simulink model "balancingOptTauExternalFsmForStep"  (Simulink 8.3)
settings: Solver=FixedStepDiscrete  StartTime=0.0  StopTime=simulationTime  FixedStep=Ts  RelTol=1e-3
InitFcn:
  | initBalancingOptTauExternalFsmForStep;
values from neighbouring files (symbols this model uses):
  localName = 'matlabTorqueBalancing'    [initBalancingOptTauExternalFsmForStep.m]
  Ts = 0.01    [initBalancingOptTauExternalFsmForStep.m]
undefined symbols (not defined in the file or in its folder): dampings, DiscIntNeverNeededParam, forceThreshold, gainMomentum, gainsDCOM, gainsICOM, gainsPCOM, impedances, impedencesSat, increasingRatesImp, qTildeMax, ROBOT_DOF_FOR_SIMULINK
undefined symbols (not defined in the file): robotName
libraries: WBCLibrary x45
settings Model: Creator=daniele  LastModifiedBy=daniele
settings DataIOCC: SignalLoggingSaveFormat=Dataset
settings OptimizationCC: ExpressionDepthLimit=2147483647
settings DebuggingCC: FcnCallInpInsideContextMsg=EnableAllAsWarning
settings SFSimCC: SimParseCustomCode=off

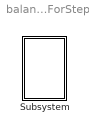
== system balancingOptTauExternalFsmForStep ==
  Subsystem : Subsystem  mask{robotName=robotName, Ts=Ts, localName=localName}
      mask prompts: robotName "robot name"; localName "module name"

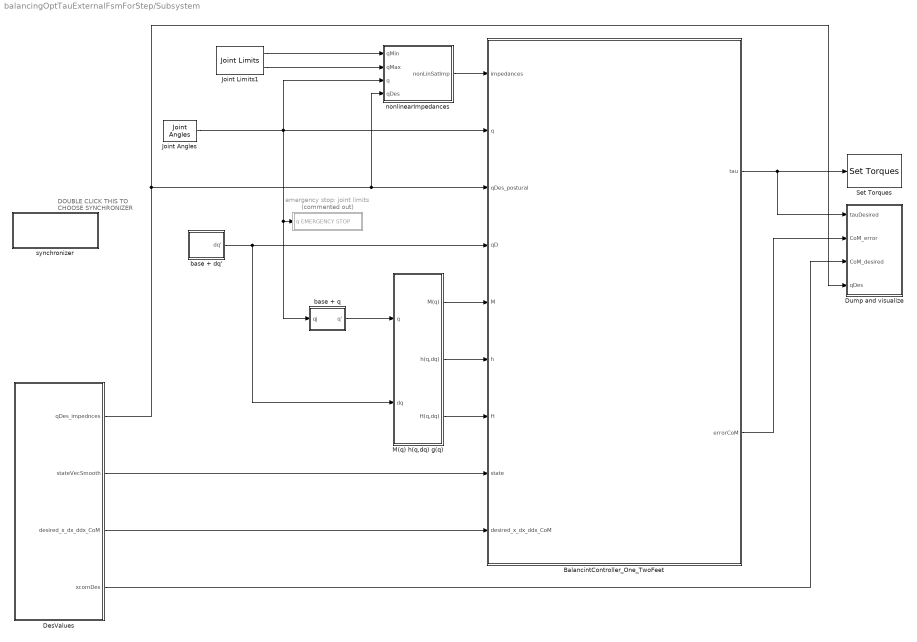
== system balancingOptTauExternalFsmForStep/Subsystem ==
  note: DOUBLE CLICK THIS TO
      |  CHOOSE SYNCHRONIZER
  BalancintController_One_TwoFeet : Subsystem
  DesValues : Subsystem
  Dump and visualize : Subsystem
  Joint Angles : WBCLibrary/wholeBodyStates/Joint Angles  robotName=robotName  localName=localName
  Joint Limits1 : WBCLibrary/wholeBodyModel/Joint Limits  robotName=robotName  localName=localName
  M(q) h(q,dq) g(q) : Subsystem
  Set Torques : WBCLibrary/wholeBodyActuators/Set Torques  val=6  robotName=robotName  localName=localName
  base + dq' : Subsystem
  base + q : Subsystem
  emergency stop: joint limits : Subsystem  Commented=on
  nonlinearImpedances : Subsystem
  synchronizer : Subsystem
  wires:
  base + q/1(q') -> M(q) h(q,dq) g(q)/1(q)
  M(q) h(q,dq) g(q)/3(H(q,dq)) -> BalancintController_One_TwoFeet/7(H)
  base + dq'/1(dq') -> M(q) h(q,dq) g(q)/2(dq), BalancintController_One_TwoFeet/4(qD)
  M(q) h(q,dq) g(q)/1(M(q)) -> BalancintController_One_TwoFeet/5(M)
  M(q) h(q,dq) g(q)/2(h(q,dq)) -> BalancintController_One_TwoFeet/6(h)
  BalancintController_One_TwoFeet/1(tau) -> Set Torques/1, Dump and visualize/1(tauDesired)
  BalancintController_One_TwoFeet/2(errorCoM) -> Dump and visualize/2(CoM_error)
  DesValues/4(xcomDes) -> Dump and visualize/3(CoM_desired)
  DesValues/3(desired_x_dx_ddx_CoM) -> BalancintController_One_TwoFeet/9(desired_x_dx_ddx_CoM)
  nonlinearImpedances/1(nonLinSatImp) -> BalancintController_One_TwoFeet/1(impedances)
  DesValues/2(stateVecSmooth) -> BalancintController_One_TwoFeet/8(state)
  DesValues/1(qDes_impednces) -> Dump and visualize/4(qDes), nonlinearImpedances/4(qDes), BalancintController_One_TwoFeet/3(qDes_postural)
  Joint Limits1/1 -> nonlinearImpedances/1(qMin)
  Joint Limits1/2 -> nonlinearImpedances/2(qMax)
  Joint Angles/1 -> nonlinearImpedances/3(q), base + q/1(qj), emergency stop: joint limits/1(q EMERGENCY STOP), BalancintController_One_TwoFeet/2(q)

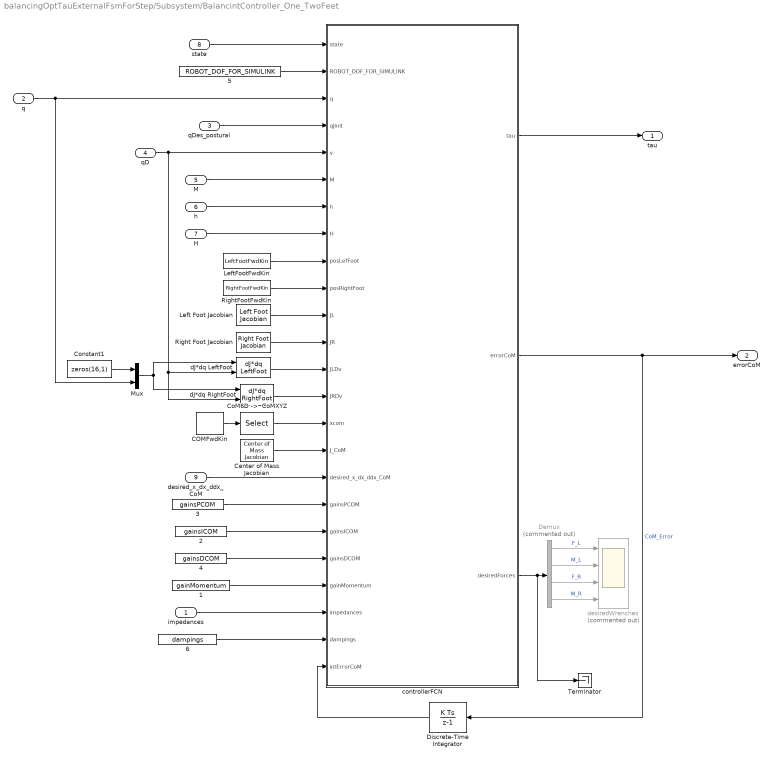
== system balancingOptTauExternalFsmForStep/Subsystem/BalancintController_One_TwoFeet ==
  impedances : Inport
  q : Inport  Port=2
  qDes_postural : Inport  Port=3
  qD : Inport  Port=4
  M : Inport  Port=5
  h : Inport  Port=6
  H : Inport  Port=7
  state : Inport  Port=8
  desired_x_dx_ddx_CoM : Inport  Port=9
  "    1" : Constant  Value=gainMomentum
  "    2" : Constant  Value=gainsICOM
  "    3" : Constant  Value=gainsPCOM
  "    4" : Constant  Value=gainsDCOM
  "    5" : Constant  Value=ROBOT_DOF_FOR_SIMULINK
  "    6" : Constant  Value=dampings
  "COMFwdKin " : WBCLibrary/wholeBodyModel/Forward Kinematics/COMFwdKin   robotName=robotName  localName=localName
  Center of Mass Jacobian : WBCLibrary/wholeBodyModel/Jacobians/Center of Mass Jacobian  robotName=robotName  localName=localName
  "CoM6D ->  CoMXYZ" : Selector  InputPortWidth=7  Indices=[1 2 3]
  Constant1 : Constant  Value=zeros(16,1)
  Demux : Demux  Commented=on
  Discrete-Time Integrator : DiscreteIntegrator  InitialCondition=[0 0 0]  SampleTime=Ts  ICPrevOutput=DiscIntNeverNeededParam  ICPrevScaledInput=DiscIntNeverNeededParam
  Left Foot Jacobian : WBCLibrary/wholeBodyModel/Jacobians/Left Foot Jacobian  robotName=robotName  localName=localName
  LeftFootFwdKin : WBCLibrary/wholeBodyModel/Forward Kinematics/LeftFootFwdKin  robotName=robotName  localName=localName
  Mux : Mux  Inputs=2
  Right Foot Jacobian : WBCLibrary/wholeBodyModel/Jacobians/Right Foot Jacobian  robotName=robotName  localName=localName
  RightFootFwdKin : WBCLibrary/wholeBodyModel/Forward Kinematics/RightFootFwdKin  robotName=robotName  localName=localName
  Terminator : Terminator
  controllerFCN : MATLAB Function  TreatAsAtomicUnit=on
  dJ*dq LeftFoot : WBCLibrary/wholeBodyModel/Dynamics/dJ*dq LeftFoot  val=9  robotName=robotName  localName=localName
  dJ*dq RightFoot : WBCLibrary/wholeBodyModel/Dynamics/dJ*dq RightFoot  val=9  robotName=robotName  localName=localName
  desiredWrenches : Scope  Commented=on  NumInputPorts=4
      settings: ShowLegends=on  TimeRange=150  YMin=-5~-5~63.70967741935465~-5  YMax=5~5~150~5  SaveName=ScopeData2
  tau : Outport
  errorCoM : Outport  Port=2
  wires:
  q/1 -> Mux/2, controllerFCN/3(q)
  qDes_postural/1 -> controllerFCN/4(qjInit)
  qD/1 -> dJ*dq RightFoot/2, dJ*dq LeftFoot/2, controllerFCN/5(v)
  M/1 -> controllerFCN/6(M)
  h/1 -> controllerFCN/7(h)
  H/1 -> controllerFCN/8(H)
  Left Foot Jacobian/1 -> controllerFCN/11(JL)
  Right Foot Jacobian/1 -> controllerFCN/12(JR)
  desired_x_dx_ddx_CoM/1 -> controllerFCN/17(desired_x_dx_ddx_CoM)
  impedances/1 -> controllerFCN/22(impedances)
  Discrete-Time Integrator/1 -> controllerFCN/24(intErrorCoM)
  "    3"/1 -> controllerFCN/18(gainsPCOM)
  "    1"/1 -> controllerFCN/21(gainMomentum)
  "    2"/1 -> controllerFCN/19(gainsICOM)
  "    4"/1 -> controllerFCN/20(gainsDCOM)
  controllerFCN/1(tau) -> tau/1
  "    5"/1 -> controllerFCN/2(ROBOT_DOF_FOR_SIMULINK)
  "    6"/1 -> controllerFCN/23(dampings)
  controllerFCN/3(desiredForces) -> Terminator/1, Demux/1
  Demux/1 -> desiredWrenches/1  "F_L"
  Demux/2 -> desiredWrenches/2  "M_L"
  Demux/3 -> desiredWrenches/3  "F_R"
  Demux/4 -> desiredWrenches/4  "M_R"
  state/1 -> controllerFCN/1(state)
  dJ*dq LeftFoot/1 -> controllerFCN/13(JLDv)
  dJ*dq RightFoot/1 -> controllerFCN/14(JRDv)
  Constant1/1 -> Mux/1
  Mux/1 -> dJ*dq RightFoot/1, dJ*dq LeftFoot/1
  "COMFwdKin "/1 -> "CoM6D ->  CoMXYZ"/1
  "CoM6D ->  CoMXYZ"/1 -> controllerFCN/15(xcom)
  RightFootFwdKin/1 -> controllerFCN/10(posRightFoot)
  Center of Mass Jacobian/1 -> controllerFCN/16(J_CoM)
  LeftFootFwdKin/1 -> controllerFCN/9(posLefFoot)
  controllerFCN/2(errorCoM) -> Discrete-Time Integrator/1, errorCoM/1  "CoM_Error"

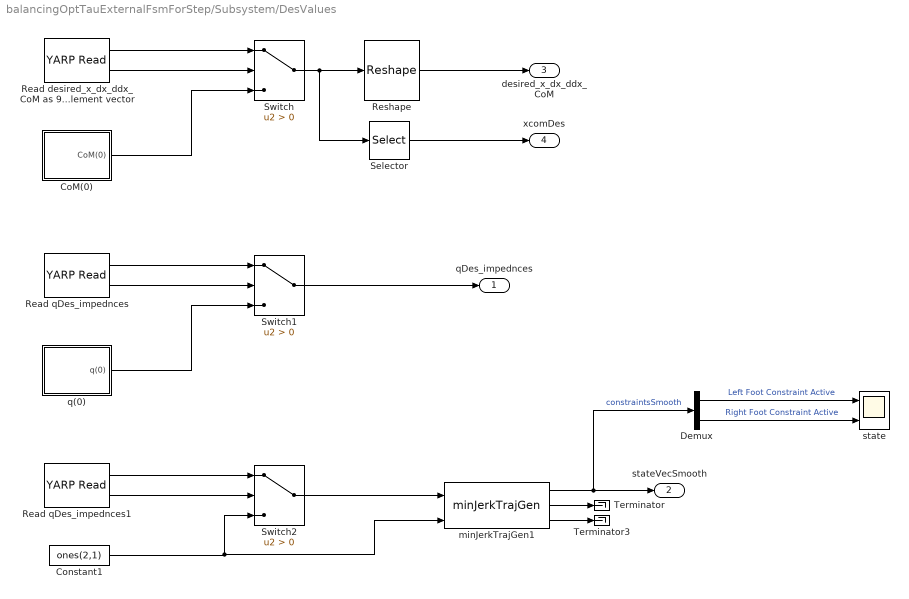
== system balancingOptTauExternalFsmForStep/Subsystem/DesValues ==
  CoM(0) : Subsystem
  Constant1 : Constant  Value=ones(2,1)
  Demux : Demux  Outputs=2
  "Read desired_x_dx_ddx_CoM as 9 element vector " : WBCLibrary/Utilities/YARP Read  portName=['/' localName '/comDes:i']  signalSize=9  blocking=off  timestamp=off  autoconnect=off
  Read qDes_impednces : WBCLibrary/Utilities/YARP Read  portName=['/' localName '/qDes:i']  signalSize=ROBOT_DOF  blocking=off  timestamp=off  autoconnect=off
  Read qDes_impednces1 : WBCLibrary/Utilities/YARP Read  portName=['/' localName '/constraints:i']  signalSize=2  blocking=off  timestamp=off  autoconnect=off
  Reshape : Reshape  OutputDimensionality=Customize  OutputDimensions=[3,3]
  Selector : Selector  InputPortWidth=9  Indices=[1:3]
  Switch : Switch  Criteria=u2 > Threshold
  Switch1 : Switch  Criteria=u2 > Threshold
  Switch2 : Switch  Criteria=u2 > Threshold
  Terminator : Terminator
  Terminator3 : Terminator
  minJerkTrajGen1 : WBCLibrary/Utilities/minJerkTrajGen  dim=2  Ts=Ts  Tt=smoothingTimeJacobians
  q(0) : Subsystem
  state : Scope  NumInputPorts=2
      settings: ShowLegends=on  TimeRange=120  YMin=0~0  YMax=2~2
  qDes_impednces : Outport
  stateVecSmooth : Outport  Port=2
  desired_x_dx_ddx_CoM : Outport  Port=3
  xcomDes : Outport  Port=4
  wires:
  Constant1/1 -> minJerkTrajGen1/2, Switch2/3
  minJerkTrajGen1/1 -> Demux/1, stateVecSmooth/1  "constraintsSmooth"
  minJerkTrajGen1/2 -> Terminator/1
  minJerkTrajGen1/3 -> Terminator3/1
  "Read desired_x_dx_ddx_CoM as 9 element vector "/2 -> Switch/2
  "Read desired_x_dx_ddx_CoM as 9 element vector "/1 -> Switch/1
  Reshape/1 -> desired_x_dx_ddx_CoM/1
  Switch/1 -> Selector/1, Reshape/1
  CoM(0)/1(CoM(0)) -> Switch/3
  Read qDes_impednces/2 -> Switch1/2
  Read qDes_impednces/1 -> Switch1/1
  q(0)/1(q(0)) -> Switch1/3
  Switch1/1 -> qDes_impednces/1
  Selector/1 -> xcomDes/1
  Read qDes_impednces1/2 -> Switch2/2
  Read qDes_impednces1/1 -> Switch2/1
  Switch2/1 -> minJerkTrajGen1/1
  Demux/1 -> state/1  "Left Foot Constraint Active"
  Demux/2 -> state/2  "Right Foot Constraint Active"

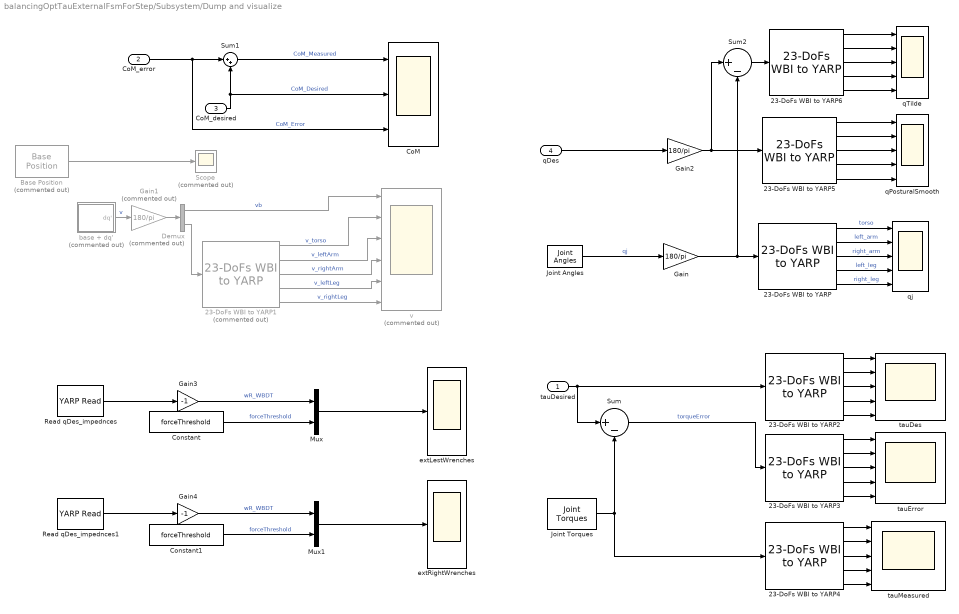
== system balancingOptTauExternalFsmForStep/Subsystem/Dump and visualize ==
  tauDesired : Inport
  CoM_error : Inport  Port=2
  CoM_desired : Inport  Port=3
  qDes : Inport  Port=4
  23-DoFs WBI to YARP{,2..6} (6 alike) : WBCLibrary/Utilities/23-DoFs WBI to YARP
  23-DoFs WBI to YARP1 : WBCLibrary/Utilities/23-DoFs WBI to YARP  Commented=on
  Base Position : WBCLibrary/wholeBodyStates/Base Position  Commented=on  robotName=robotName  localName=localName
  CoM : Scope  NumInputPorts=3
      settings: ShowLegends=on  TimeRange=30  YMin=-0.09999999999999998~-0.1~-0.011  YMax=0.55~0.6000000000000001~0.008  SaveName=CoM_data
  Constant : Constant  Value=forceThreshold
  Constant1 : Constant  Value=forceThreshold
  Demux : Demux  Commented=on  Outputs=2
  Gain : Gain  Gain=180/pi
  Gain1 : Gain  Commented=on  Gain=180/pi
  Gain2 : Gain  Gain=180/pi
  Gain3 : Gain  Gain=-1
  Gain4 : Gain  Gain=-1
  Joint Angles : WBCLibrary/wholeBodyStates/Joint Angles  robotName=robotName  localName=localName
  Joint Torques : WBCLibrary/wholeBodyStates/Joint Torques  robotName=robotName  localName=localName
  Mux : Mux  Inputs=2
  Mux1 : Mux  Inputs=2
  Read qDes_impednces : WBCLibrary/Utilities/YARP Read  portName=['/wholeBodyDynamicsTree/left_leg/endEffectorWrench:o']  signalSize=6  blocking=off  timestamp=off  autoconnect=on
  Read qDes_impednces1 : WBCLibrary/Utilities/YARP Read  portName='/wholeBodyDynamicsTree/right_leg/endEffectorWrench:o'  signalSize=6  blocking=off  timestamp=off  autoconnect=on
  Scope : Scope  Commented=on
      settings: ShowLegends=on  SaveName=ScopeData4
  Sum : Sum  Inputs=|+-
  Sum1 : Sum  Inputs=|++
  Sum2 : Sum  Inputs=|+-
  base + dq' : Subsystem  Commented=on
  extLestWrenches : Scope
      settings: ShowLegends=on  TimeRange=0.1833217047788445  YMin=13.8828873386089  YMax=21.49690233236151
  extRightWrenches : Scope
      settings: ShowLegends=on  TimeRange=0.1833217047788445  YMin=13.8828873386089  YMax=21.49690233236151  SaveName=ScopeData6
  qPosturalSmooth : Scope  NumInputPorts=5
      settings: ShowLegends=on  TimeRange=34.19  YMin=-1e-27~-40~-40~-20~-20  YMax=1e-28~60~60~20~20  SaveName=ScopeData3
  qTilde : Scope  NumInputPorts=5
      settings: ShowLegends=on  TimeRange=120  YMin=-20~-30~-30~-20~-4  YMax=40~30~30~10~4  SaveName=ScopeData5
  qj : Scope  NumInputPorts=5
      settings: ShowLegends=on  TimeRange=400  YMin=-40~-50~-50~-20~-40  YMax=20~100~100~40~40  SaveName=qj_and_v
  tauDes : Scope  NumInputPorts=5
      settings: ShowLegends=on  TimeRange=22.09  YMin=-30~-4~-10~-10~-10  YMax=10~4~5~10~10  SaveName=tauDes
  tauError : Scope  NumInputPorts=5
      settings: ShowLegends=on  TimeRange=18.63  YMin=-1~-1~-1~-10~-10  YMax=2~1~1~15~15  SaveName=tauError
  tauMeasured : Scope  NumInputPorts=5
      settings: ShowLegends=on  TimeRange=30  YMin=-6~-4~-4~-10~-10  YMax=2~2~2~30~10  SaveName=tauMeasured
  v : Scope  Commented=on  NumInputPorts=6
      settings: ShowLegends=on  TimeRange=10  YMin=-0.124~-5~-5~-5~-5~-5  YMax=-0.106~5~5~5~5~5  SaveName=qj_and_v1
  wires:
  CoM_error/1 -> CoM/3, Sum1/1  "CoM_Error"
  tauDesired/1 -> 23-DoFs WBI to YARP2/1, Sum/1
  23-DoFs WBI to YARP3/3 -> tauError/3
  23-DoFs WBI to YARP2/4 -> tauDes/4
  23-DoFs WBI to YARP3/4 -> tauError/4
  23-DoFs WBI to YARP2/3 -> tauDes/3
  23-DoFs WBI to YARP4/4 -> tauMeasured/4
  23-DoFs WBI to YARP3/1 -> tauError/1
  23-DoFs WBI to YARP4/5 -> tauMeasured/5
  Joint Torques/1 -> 23-DoFs WBI to YARP4/1, Sum/2
  23-DoFs WBI to YARP4/3 -> tauMeasured/3
  23-DoFs WBI to YARP4/2 -> tauMeasured/2
  CoM_desired/1 -> Sum1/2, CoM/2  "CoM_Desired"
  23-DoFs WBI to YARP3/2 -> tauError/2
  23-DoFs WBI to YARP4/1 -> tauMeasured/1
  Sum1/1 -> CoM/1  "CoM_Measured"
  23-DoFs WBI to YARP3/5 -> tauError/5
  23-DoFs WBI to YARP2/1 -> tauDes/1
  Sum/1 -> 23-DoFs WBI to YARP3/1  "torqueError"
  23-DoFs WBI to YARP2/2 -> tauDes/2
  23-DoFs WBI to YARP2/5 -> tauDes/5
  base + dq'/1(dq') -> Gain1/1  "v"
  Joint Angles/1 -> Gain/1  "qj"
  Gain/1 -> Sum2/2, 23-DoFs WBI to YARP/1
  23-DoFs WBI to YARP/5 -> qj/5  "right_leg"
  23-DoFs WBI to YARP/1 -> qj/1  "torso"
  23-DoFs WBI to YARP/2 -> qj/2  "left_arm"
  23-DoFs WBI to YARP/4 -> qj/4  "left_leg"
  23-DoFs WBI to YARP/3 -> qj/3  "right_arm"
  Gain1/1 -> Demux/1
  Demux/2 -> 23-DoFs WBI to YARP1/1
  23-DoFs WBI to YARP1/5 -> v/6  "v_rightLeg"
  23-DoFs WBI to YARP1/4 -> v/5  "v_leftLeg"
  23-DoFs WBI to YARP1/3 -> v/4  "v_rightArm"
  23-DoFs WBI to YARP1/2 -> v/3  "v_leftArm"
  23-DoFs WBI to YARP1/1 -> v/2  "v_torso"
  Demux/1 -> v/1  "vb"
  23-DoFs WBI to YARP5/3 -> qPosturalSmooth/3
  23-DoFs WBI to YARP5/1 -> qPosturalSmooth/1
  23-DoFs WBI to YARP5/2 -> qPosturalSmooth/2
  23-DoFs WBI to YARP5/4 -> qPosturalSmooth/4
  Gain2/1 -> Sum2/1, 23-DoFs WBI to YARP5/1
  qDes/1 -> Gain2/1
  23-DoFs WBI to YARP5/5 -> qPosturalSmooth/5
  23-DoFs WBI to YARP6/3 -> qTilde/3
  23-DoFs WBI to YARP6/1 -> qTilde/1
  23-DoFs WBI to YARP6/2 -> qTilde/2
  23-DoFs WBI to YARP6/4 -> qTilde/4
  23-DoFs WBI to YARP6/5 -> qTilde/5
  Sum2/1 -> 23-DoFs WBI to YARP6/1
  Mux/1 -> extLestWrenches/1
  Constant/1 -> Mux/2  "forceThreshold"
  Read qDes_impednces/1 -> Gain3/1
  Gain3/1 -> Mux/1  "wR_WBDT"
  Base Position/1 -> Scope/1
  Mux1/1 -> extRightWrenches/1
  Constant1/1 -> Mux1/2  "forceThreshold"
  Read qDes_impednces1/1 -> Gain4/1
  Gain4/1 -> Mux1/1  "wR_WBDT"

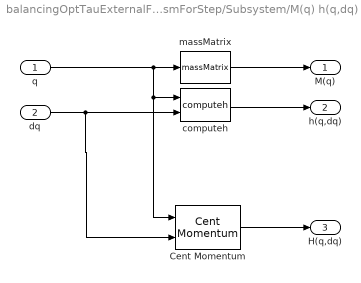
== system balancingOptTauExternalFsmForStep/Subsystem/M(q) h(q,dq) g(q) ==
  q : Inport
  dq : Inport  Port=2
  Cent Momentum : WBCLibrary/wholeBodyModel/Dynamics/Cent Momentum  robotName=robotName  localName=localName
  computeh : WBCLibrary/wholeBodyModel/Dynamics/computeh  val=7  robotname=robotName  localname=localName
  massMatrix : WBCLibrary/wholeBodyModel/Dynamics/massMatrix  val=8  robotname=robotName  localname=localName
  M(q) : Outport
  h(q,dq) : Outport  Port=2
  H(q,dq) : Outport  Port=3
  wires:
  computeh/1 -> h(q,dq)/1
  massMatrix/1 -> M(q)/1
  q/1 -> Cent Momentum/1, computeh/1, massMatrix/1
  dq/1 -> Cent Momentum/2, computeh/2
  Cent Momentum/1 -> H(q,dq)/1

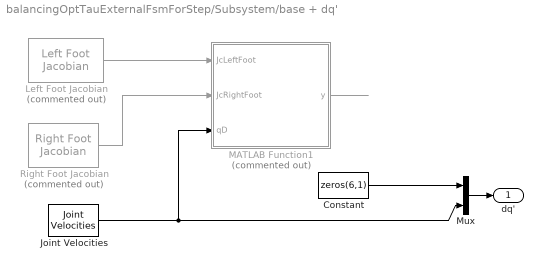
== system balancingOptTauExternalFsmForStep/Subsystem/base + dq' ==
  Constant : Constant  Value=zeros(6,1)
  Joint Velocities : WBCLibrary/wholeBodyStates/Joint Velocities  robotName=robotName  localName=localName
  Left Foot Jacobian : WBCLibrary/wholeBodyModel/Jacobians/Left Foot Jacobian  Commented=on  robotName=robotName  localName=localName
  MATLAB Function1 : MATLAB Function  Commented=on  TreatAsAtomicUnit=on
  Mux : Mux  Inputs=2
  Right Foot Jacobian : WBCLibrary/wholeBodyModel/Jacobians/Right Foot Jacobian  Commented=on  robotName=robotName  localName=localName
  dq' : Outport
  wires:
  Left Foot Jacobian/1 -> MATLAB Function1/1(JcLeftFoot)
  MATLAB Function1/1(y) -> ?
  Mux/1 -> dq'/1
  Right Foot Jacobian/1 -> MATLAB Function1/2(JcRightFoot)
  Joint Velocities/1 -> Mux/2, MATLAB Function1/3(qD)
  Constant/1 -> Mux/1

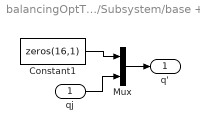
== system balancingOptTauExternalFsmForStep/Subsystem/base + q ==
  qj : Inport
  Constant1 : Constant  Value=zeros(16,1)
  Mux : Mux  Inputs=2
  q' : Outport
  wires:
  Mux/1 -> q'/1
  qj/1 -> Mux/2
  Constant1/1 -> Mux/1

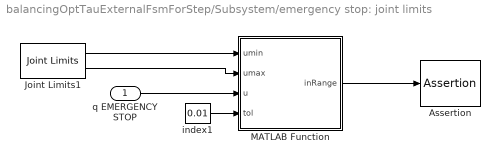
== system balancingOptTauExternalFsmForStep/Subsystem/emergency stop: joint limits ==
  q EMERGENCY STOP : Inport
  Assertion : Assertion
  Joint Limits1 : WBCLibrary/wholeBodyModel/Joint Limits  robotName=robotName  localName=localName
  MATLAB Function : MATLAB Function  TreatAsAtomicUnit=on
  index1 : Constant  Value=0.01  VectorParams1D=off
  wires:
  Joint Limits1/1 -> MATLAB Function/1(umin)
  Joint Limits1/2 -> MATLAB Function/2(umax)
  index1/1 -> MATLAB Function/4(tol)
  q EMERGENCY STOP/1 -> MATLAB Function/3(u)
  MATLAB Function/1(inRange) -> Assertion/1

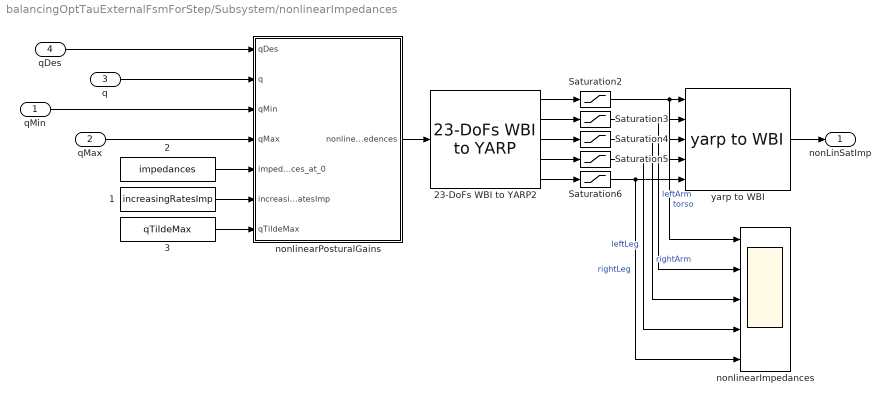
== system balancingOptTauExternalFsmForStep/Subsystem/nonlinearImpedances ==
  qMin : Inport
  qMax : Inport  Port=2
  q : Inport  Port=3
  qDes : Inport  Port=4
  "    1" : Constant  Value=increasingRatesImp
  "    2" : Constant  Value=impedances
  "    3" : Constant  Value=qTildeMax
  23-DoFs WBI to YARP2 : WBCLibrary/Utilities/23-DoFs WBI to YARP
  Saturation2 : Saturate  UpperLimit=impedencesSat(1)  LowerLimit=0  SampleTime=Ts
  Saturation3 : Saturate  UpperLimit=impedencesSat(2)  LowerLimit=0  SampleTime=Ts
  Saturation4 : Saturate  UpperLimit=impedencesSat(2)  LowerLimit=0  SampleTime=Ts
  Saturation5 : Saturate  UpperLimit=impedencesSat(3)  LowerLimit=0  SampleTime=Ts
  Saturation6 : Saturate  UpperLimit=impedencesSat(3)  LowerLimit=0  SampleTime=Ts
  nonlinearImpedances : Scope  NumInputPorts=5
      settings: ShowLegends=on  TimeRange=25  YMin=-50~-50~-50~0~0  YMax=50~50~50~1000~1000
  "nonlinearPosturalGains " : MATLAB Function  TreatAsAtomicUnit=on
  yarp to WBI : WBCLibrary/Utilities/yarp to WBI
  nonLinSatImp : Outport
  wires:
  23-DoFs WBI to YARP2/1 -> Saturation2/1
  23-DoFs WBI to YARP2/2 -> Saturation3/1
  23-DoFs WBI to YARP2/3 -> Saturation4/1
  23-DoFs WBI to YARP2/5 -> Saturation6/1
  "nonlinearPosturalGains "/1(nonlinearImpedences) -> 23-DoFs WBI to YARP2/1
  qMin/1 -> "nonlinearPosturalGains "/3(qMin)
  qMax/1 -> "nonlinearPosturalGains "/4(qMax)
  "    2"/1 -> "nonlinearPosturalGains "/5(impedences_at_0)
  "    1"/1 -> "nonlinearPosturalGains "/6(increasingRatesImp)
  q/1 -> "nonlinearPosturalGains "/2(q)
  Saturation6/1 -> nonlinearImpedances/5, yarp to WBI/5  "rightLeg"
  Saturation4/1 -> nonlinearImpedances/3, yarp to WBI/3  "rightArm"
  Saturation5/1 -> nonlinearImpedances/4, yarp to WBI/4  "leftLeg"
  Saturation3/1 -> nonlinearImpedances/2, yarp to WBI/2  "leftArm"
  Saturation2/1 -> nonlinearImpedances/1, yarp to WBI/1  "torso"
  23-DoFs WBI to YARP2/4 -> Saturation5/1
  "    3"/1 -> "nonlinearPosturalGains "/7(qTildeMax)
  yarp to WBI/1 -> nonLinSatImp/1
  qDes/1 -> "nonlinearPosturalGains "/1(qDes)

== system balancingOptTauExternalFsmForStep/Subsystem/synchronizer ==
  Real Time Synchronizer : WBCLibrary/Utilities/Real Time Synchronizer  threadPeriod=Ts
  synchronize : WBCLibrary/Utilities/synchronize  Commented=on  rate=0.010  scaleFactor=1

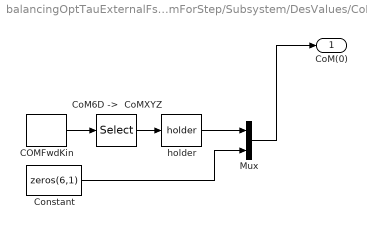
== system balancingOptTauExternalFsmForStep/Subsystem/DesValues/CoM(0) ==
  "COMFwdKin " : WBCLibrary/wholeBodyModel/Forward Kinematics/COMFwdKin   robotName=robotName  localName=localName
  "CoM6D ->  CoMXYZ" : Selector  InputPortWidth=7  Indices=[1 2 3]
  Constant : Constant  Value=zeros(6,1)
  Mux : Mux  Inputs=2
  "holder " : WBCLibrary/Utilities/holder 
  CoM(0) : Outport
  wires:
  "holder "/1 -> Mux/1
  "COMFwdKin "/1 -> "CoM6D ->  CoMXYZ"/1
  "CoM6D ->  CoMXYZ"/1 -> "holder "/1
  Mux/1 -> CoM(0)/1
  Constant/1 -> Mux/2

== system balancingOptTauExternalFsmForStep/Subsystem/DesValues/q(0) ==
  Joint Angles : WBCLibrary/wholeBodyStates/Joint Angles  robotName=robotName  localName=localName
  holder 1 : WBCLibrary/Utilities/holder 
  q(0) : Outport
  wires:
  Joint Angles/1 -> holder 1/1
  holder 1/1 -> q(0)/1

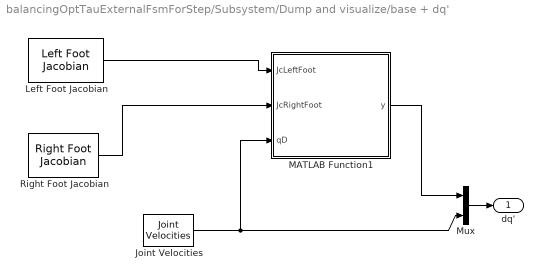
== system balancingOptTauExternalFsmForStep/Subsystem/Dump and visualize/base + dq' ==
  Joint Velocities : WBCLibrary/wholeBodyStates/Joint Velocities  robotName=robotName  localName=localName
  Left Foot Jacobian : WBCLibrary/wholeBodyModel/Jacobians/Left Foot Jacobian  robotName=robotName  localName=localName
  MATLAB Function1 : MATLAB Function  TreatAsAtomicUnit=on
  Mux : Mux  Inputs=2
  Right Foot Jacobian : WBCLibrary/wholeBodyModel/Jacobians/Right Foot Jacobian  robotName=robotName  localName=localName
  dq' : Outport
  wires:
  Left Foot Jacobian/1 -> MATLAB Function1/1(JcLeftFoot)
  MATLAB Function1/1(y) -> Mux/1
  Mux/1 -> dq'/1
  Right Foot Jacobian/1 -> MATLAB Function1/2(JcRightFoot)
  Joint Velocities/1 -> MATLAB Function1/3(qD), Mux/2

== matlab function Subsystem/base + dq'/MATLAB Function1 ==
  data: JcLeftFoot input double; JcRightFoot input double; y output double; qD input double; stateSmooth data_store_memory double
function y = fcn(JcLeftFoot,JcRightFoot,qD)
%#codegen
global stateSmooth;

Jc = [JcLeftFoot;JcRightFoot*(1-stateSmooth(3))];

y = -pinv(Jc(:,1:6))*Jc(:,7:end)*qD;

== matlab function Subsystem/BalancintController_One_TwoFeet/controllerFCN ==
  data: state input double; ROBOT_DOF_FOR_SIMULINK input double; q input double; tau output double; qjInit input double; v input double; M input double; h input double; H input double; posLefFoot input double; posRightFoot input double; JL input double; JR input double; JLDv input double; JRDv input double; xcom input double; J_CoM input double; desired_x_dx_ddx_CoM input double; gainsPCOM input double; gainsICOM input double; gainsDCOM input double; gainMomentum input double; impedances input double; dampings input double; intErrorCoM input double; errorCoM output double; desiredForces output double
function [tau,errorCoM,desiredForces]   =  controllerFCN(state,ROBOT_DOF_FOR_SIMULINK,q,qjInit,v, M, h, H, posLefFoot, posRightFoot, JL,JR, JLDv,JRDv, xcom,J_CoM, desired_x_dx_ddx_CoM, gainsPCOM,gainsICOM,gainsDCOM,gainMomentum, impedances,dampings, intErrorCoM)
%#codegen

desiredForces   = zeros(12,1);
ROBOT_DOF       = size(ROBOT_DOF_FOR_SIMULINK,1);
PINV_TOL        = 1e-5;
reg             = 0.01;
gravAcc         = 9.81;
m               = M(1,1);
Mb              = M(1:6,1:6);
Mbj             = M(1:6,7:end);
% Mj              = M(7:end,7:end);

St              = [  zeros(6,ROBOT_DOF);
                   eye(ROBOT_DOF,ROBOT_DOF)];
grav            = [ zeros(2,1);
                   -m*gravAcc;
                    zeros(3,1)];
pos_rightFoot   = posRightFoot(1:3);
pos_leftFoot    = posLefFoot(1:3);

xDcom           = J_CoM(1:3,:)*v;
qD              = v(7:end);
xDDcomStar      = desired_x_dx_ddx_CoM(:,3) - gainsPCOM*(xcom - desired_x_dx_ddx_CoM(:,1)) - gainsICOM*intErrorCoM - gainsDCOM*(xDcom - desired_x_dx_ddx_CoM(:,2));
Pr              = pos_rightFoot - xcom; % Application point of the contact force on the right foot w.r.t. CoM
Pl              = pos_leftFoot  - xcom; % Application point of the contact force on the left foot w.r.t. CoM


AL = [ eye(3),   zeros(3);
       Sf(Pl),  eye(3)];
AR = [ eye(3), zeros(3);
        Sf(Pr), eye(3) ];
    
A    = [ AL, AR];

Jc   = [ JL*state(1) ;
         JR*state(2)];
JcDv = [ JLDv*state(1) ;
         JRDv*state(2)];

JcMinv          = Jc/M;
JcMinvSt        = JcMinv*St;
JcMinvJct       = JcMinv*transpose(Jc);

pinvA         = pinv( A, PINV_TOL)*state(1)*state(2) + [inv(AL);zeros(6)]*state(1)*(1-state(2)) + [zeros(6);inv(AR)]*state(2)*(1-state(1)); 
% PInv_JcMinvSt = pinv( JcMinvSt, PINV_TOL);
PInv_JcMinvSt = JcMinvSt'/(JcMinvSt*JcMinvSt' + reg*eye(size(JcMinvSt,1)));
  
HDotDes  = [ m*xDDcomStar ;
            -gainMomentum*H(4:end)]; 
         
%% QP FOR TORQUE MINIMIZATION BASED ON arbitrary vector F0
% Maux = [     eye(3)     zeros(3,22)
%           zeros(22,3)      inv(Mj(4:end,4:end))];
%define tau_0 (the arbitrary vector)
N0_tau        = eye(ROBOT_DOF) - PInv_JcMinvSt*JcMinvSt;

mult_f_tau0   =  Mbj'/Mb*transpose(Jc(:,1:6))-transpose(Jc(:,7:end)); % multiplier of f in tau0
n_tau0        =  h(7:end) - Mbj'/Mb*h(1:6) - diag(impedances)*(q-qjInit)  -diag(dampings)*N0_tau*qD ; % additional terms in tau0 - Mj*(kPandD_Postural(1,:)'.*(q-qjInit) + kPandD_Postural(2,:)'.*qD) 
%

mult_f_tau    = -PInv_JcMinvSt*JcMinvJct    + N0_tau*mult_f_tau0;

% f desired is given as:
% f*   = pinvA*(HDotDes - grav)  + (I-pinvA*A) * f0
% f*   =           f_HDot        +     N0_f    * f0
f_HDot = pinvA*(HDotDes - grav);

% tau is given as:
% tau = (mult_f_tau*N0_f)* f0 + (n_tau+mult_f_tau*f_HDot)
% tau =        X_tau     * f0 +                   Y_tau

Y_tau            = PInv_JcMinvSt*(JcMinv*h-JcDv) + N0_tau*n_tau0 + mult_f_tau*f_HDot;

N0_f             =  eye(12,12)-pinvA*A;
X_tau            = mult_f_tau*N0_f;
if state(1) > 0.99 && state(2) > 0.99
    f0 = -pinv(X_tau, PINV_TOL)*Y_tau;
else
    f0 = zeros(12,1);
end
tau              = X_tau   * f0*state(1)*state(2)   +  Y_tau;
desiredForces    = N0_f    * f0*state(1)*state(2)   +  f_HDot;

errorCoM = xcom - desired_x_dx_ddx_CoM(:,1);

== matlab function Subsystem/emergency stop: joint limits/MATLAB Function ==
  data: umin input double; umax input double; u input double; inRange output double; tol input double
function inRange = checkRange(umin, umax, u, tol)
%#codegen

res = u < umin + tol | u > umax - tol;
res = sum(res);
if res==0
    inRange = 1;
else
    inRange = 0;
    u < umin + tol | u > umax - tol
end

== matlab function Subsystem/Dump and visualize/base + dq'/MATLAB Function1 ==
  data: JcLeftFoot input double; JcRightFoot input double; y output double; qD input double; stateSmooth data_store_memory double
function y = fcn(JcLeftFoot,JcRightFoot,qD)
%#codegen
global stateSmooth;

Jc = [JcLeftFoot;JcRightFoot*(1-stateSmooth(3))];

y = -pinv(Jc(:,1:6))*Jc(:,7:end)*qD;

== matlab function Subsystem/nonlinearImpedances/nonlinearPosturalGains  ==
  data: qDes input double; nonlinearImpedences output double; q input double; qMin input double; qMax input double; impedences_at_0 input double; increasingRatesImp input double; qTildeMax input double
function nonlinearImpedences = fcn(qDes,q,qMin,qMax,impedences_at_0,increasingRatesImp,qTildeMax)
    %#codegen

    tp =  pi./(2*(qMax-qDes));
    tn = -pi./(2*(qMin-qDes));

    
    qTilde = q - qDes;
            
    nonlinearImpedences = (impedences_at_0   + increasingRatesImp.*tan(pi.*qTilde./(2*qTildeMax)).^2)';
%                                                increasingRatesImp.*tan((tp.*stepFcn(qTilde) + tn.*stepFcn(-qTilde)).*qTilde).^2)';
                                           
end

function y = stepFcn(x) 
   %#codegen
   y = x > 0; 
end
